simulink model "Q4"  (R2019b)
settings: Solver=VariableStepAuto  StartTime=0.0  StopTime=10  RelTol=1e-3
libraries: dspsrcs4 x1
settings Model: Creator=Qusay  LastModifiedBy=Qusay

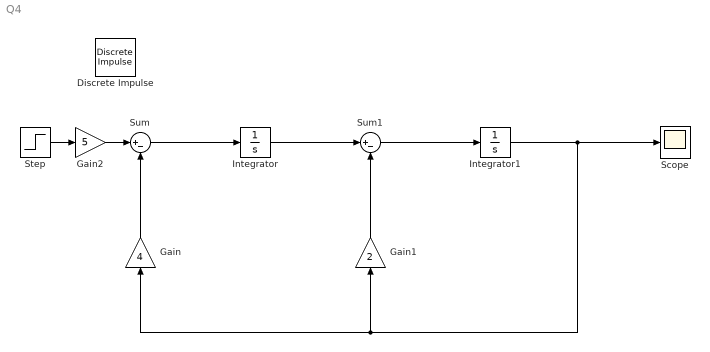
== system Q4 ==
  Discrete Impulse : dspsrcs4/Discrete  Impulse  Delay=0  SampleTime=1  FrameSample=1  OutputFrames=off  dataType=double  isSigned=on  wordLen=16  udDataType=sfix(16)  fracBitsMode=Best precision  numFracBits=15  OutDataTypeStr=double  LastOutDataTypeStr=double
  Gain : Gain  Gain=4
  Gain1 : Gain  Gain=2
  Gain2 : Gain  Gain=5
  Integrator : Integrator
  Integrator1 : Integrator
  Scope : Scope
  Step : Step  SampleTime=0
  Sum : Sum  Inputs=|+-
  Sum1 : Sum  Inputs=|+-
  wires:
  Sum/1 -> Integrator/1
  Integrator/1 -> Sum1/1
  Gain1/1 -> Sum1/2
  Sum1/1 -> Integrator1/1
  Integrator1/1 -> Gain1/1, Gain/1, Scope/1
  Gain/1 -> Sum/2
  Gain2/1 -> Sum/1
  Step/1 -> Gain2/1
